simulink model "HW2_2106A503_IVD"  (R2024b)
settings: Solver=VariableStepAuto  StartTime=0.0  StopTime=10.0  RelTol=1e-3
values from neighbouring files (symbols this model uses):
  alpha_rad = deg2rad(alpha_deg)    [HW2_TireModels.m]
undefined symbols (not defined in the file or in its folder): alpha_axis, Fx_dugoff_sim, Fx_fiala_sim, Fx_magic_sim, Fy_dugoff_sim, Fy_fiala_sim, Fy_magic_sim, fz_axis, slip_axis, slip_axis_pct
libraries: simulink x6
settings Model: Creator=Losceret  LastModifiedBy=Losceret
settings DataIOCC: ReturnWorkspaceOutputs=off

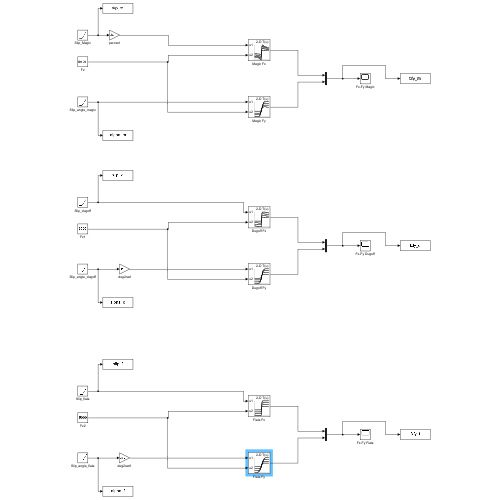
[thumbnail: Simulink's stored preview of the top-level diagram]
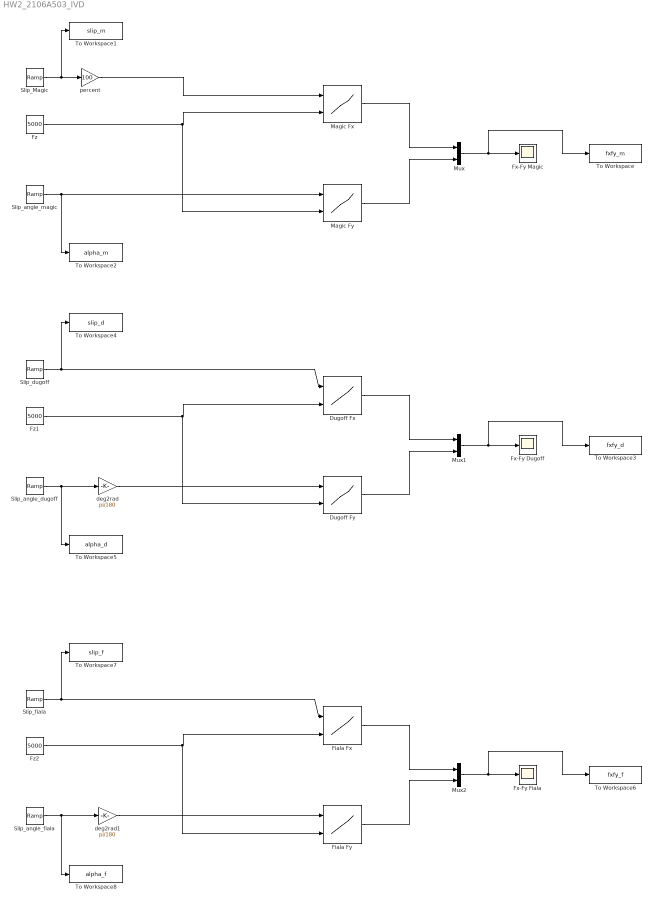
== system HW2_2106A503_IVD ==
  Dugoff Fx : Lookup_n-D  BreakpointsForDimension1=slip_axis  BreakpointsForDimension2=fz_axis  Table=Fx_dugoff_sim  InternalRulePriority=Speed  RndMeth=Simplest
      settings: InputPortMap=u0,u1
  Dugoff Fy : Lookup_n-D  BreakpointsForDimension1=alpha_rad  BreakpointsForDimension2=fz_axis  Table=Fy_dugoff_sim  InternalRulePriority=Speed  RndMeth=Simplest
      settings: InputPortMap=u0,u1
  Fiala Fx : Lookup_n-D  BreakpointsForDimension1=slip_axis  BreakpointsForDimension2=fz_axis  Table=Fx_fiala_sim  InternalRulePriority=Speed  RndMeth=Simplest
      settings: InputPortMap=u0,u1
  Fiala Fy : Lookup_n-D  BreakpointsForDimension1=alpha_rad  BreakpointsForDimension2=fz_axis  Table=Fy_fiala_sim  InternalRulePriority=Speed  RndMeth=Simplest
      settings: InputPortMap=u0,u1
  Fx-Fy Dugoff : Scope
  Fx-Fy Fiala : Scope
  Fx-Fy Magic : Scope
  Fz : Constant  Value=5000
  Fz1 : Constant  Value=5000
  Fz2 : Constant  Value=5000
  Magic Fx : Lookup_n-D  BreakpointsForDimension1=slip_axis_pct  BreakpointsForDimension2=fz_axis  Table=Fx_magic_sim  InternalRulePriority=Speed  RndMeth=Simplest
      settings: InputPortMap=u0,u1
  Magic Fy : Lookup_n-D  BreakpointsForDimension1=alpha_axis  BreakpointsForDimension2=fz_axis  Table=Fy_magic_sim  InternalRulePriority=Speed  RndMeth=Simplest
      settings: InputPortMap=u0,u1
  Mux : Mux  Inputs=2
  Mux1 : Mux  Inputs=2
  Mux2 : Mux  Inputs=2
  Slip_Magic : simulink/Sources/Ramp  slope=0.2  start=0  InitialOutput=-1
  Slip_angle_dugoff : simulink/Sources/Ramp  slope=5  start=0  InitialOutput=-25
  Slip_angle_fiala : simulink/Sources/Ramp  slope=5  start=0  InitialOutput=-25
  Slip_angle_magic : simulink/Sources/Ramp  slope=5  start=0  InitialOutput=-25
  Slip_dugoff : simulink/Sources/Ramp  slope=0.2  start=0  InitialOutput=-1
  Slip_fiala : simulink/Sources/Ramp  slope=0.2  start=0  InitialOutput=-1
  To Workspace : ToWorkspace  VariableName=fxfy_m  SampleTime=-1
  To Workspace1 : ToWorkspace  VariableName=slip_m  SampleTime=-1
  To Workspace2 : ToWorkspace  VariableName=alpha_m  SampleTime=-1
  To Workspace3 : ToWorkspace  VariableName=fxfy_d  SampleTime=-1
  To Workspace4 : ToWorkspace  VariableName=slip_d  SampleTime=-1
  To Workspace5 : ToWorkspace  VariableName=alpha_d  SampleTime=-1
  To Workspace6 : ToWorkspace  VariableName=fxfy_f  SampleTime=-1
  To Workspace7 : ToWorkspace  VariableName=slip_f  SampleTime=-1
  To Workspace8 : ToWorkspace  VariableName=alpha_f  SampleTime=-1
  deg2rad : Gain  Gain=pi/180
  deg2rad1 : Gain  Gain=pi/180
  percent : Gain  Gain=100
  wires:
  Slip_Magic/1 -> To Workspace1/1, percent/1
  percent/1 -> Magic Fx/1
  Fz/1 -> Magic Fy/2, Magic Fx/2
  Slip_angle_magic/1 -> To Workspace2/1, Magic Fy/1
  Magic Fy/1 -> Mux/2
  Magic Fx/1 -> Mux/1
  Mux/1 -> To Workspace/1, Fx-Fy Magic/1
  Slip_angle_dugoff/1 -> To Workspace5/1, deg2rad/1
  Mux1/1 -> To Workspace3/1, Fx-Fy Dugoff/1
  Dugoff Fy/1 -> Mux1/2
  Dugoff Fx/1 -> Mux1/1
  Fz1/1 -> Dugoff Fy/2, Dugoff Fx/2
  Slip_dugoff/1 -> Dugoff Fx/1, To Workspace4/1
  deg2rad/1 -> Dugoff Fy/1
  Slip_angle_fiala/1 -> To Workspace8/1, deg2rad1/1
  Mux2/1 -> To Workspace6/1, Fx-Fy Fiala/1
  Fz2/1 -> Fiala Fy/2, Fiala Fx/2
  Fiala Fx/1 -> Mux2/1
  Slip_fiala/1 -> Fiala Fx/1, To Workspace7/1
  Fiala Fy/1 -> Mux2/2
  deg2rad1/1 -> Fiala Fy/1
